simulink model "IRP6"  (R2015a)
settings: Solver=ode1  StartTime=0.0  StopTime=Inf  FixedStep=0.001  RelTol=1e-3
PostLoadFcn:
  | , if any(exist('dsrtsu_mdlpostloadfcn', 'file') == [2, 3, 6]), try dsrtsu_mdlpostloadfcn('Execute', bdroot); catch fprintf('Error in PostLoadFcn (dsrtsu_mdlpostloadfcn) for model "%s":\n %s\n', bdroot, lasterr); end, end,
libraries: simulink x15, rtilibm x3
(part 1 of 2)
settings Model: DSRTSU_INTERNAL_RTI_VER=460  DSRTSU_INTERNAL_RTI_TYPE=rti1005  DSRTSU_INTERNAL_RTIFPGA=50  CovHtmlReporting=off  Creator=k22p800b  LastModifiedBy=k22p800b
settings OptimizationCC: BlockReduction=off  BooleanDataType=off  OptimizeBlockIOStorage=off  BufferReuse=off  GlobalBufferReuse=off  ExpressionFolding=off  LocalBlockOutputs=off
settings HardwareCC: ProdIntDivRoundTo=Zero  ProdEndianess=BigEndian  ProdHWDeviceType=Generic->Custom  TargetIntDivRoundTo=Zero  TargetEndianess=BigEndian  TargetHWDeviceType=Generic->Custom
settings RTWCC: SystemTargetFile=rti1005.tlc  MakeCommand=make_rti  TemplateMakefile=rti1005.tmf  Description=dSPACE DS1005 Hardware Platform
settings STFCustomTargetCC: GenerateSampleERTMain=off  ParMdlRefBuildCompliant=on  GeneratePreprocessorConditionals=Disable all  ERTCustomFileBanners=off  SupportNonInlinedSFcns=on  SupportVariableSizeSignals=off  MATLABClassNameForMDSCustomization=Simulink.SoftwareTarget.GRTCustomization  GRTInterface=on  SystemTargetFile=rti1005.tlc
settings GRTTargetCC: CompOptLevelCompliant=off  ConcurrentExecutionCompliant=off  CombineOutputUpdateFcns=off  MatFileLogging=off  CPPClassGenCompliant=off  GRTInterface=on  ExtModeMexFile=noextcomm

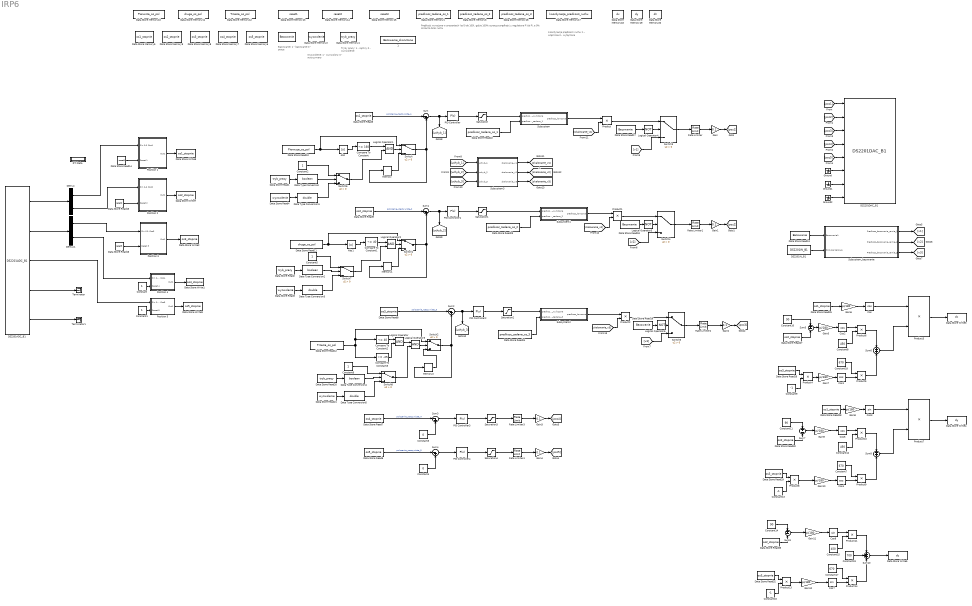
== system IRP6 ==
  note: A
  note: Bazowanie:
      | 1 - bazowanie
      | 0 - praca
  note: Tryby pracy:
      | 1 - ręczny
      | 0 - wyzwolenie
  note: Wyzwolenie:
      | 1 - wyzwolony
      | 0 - wstrzymany
  note: Prędkość wyrażona w procentach (od 0 do 100), gdzie 100% oznacza
      | prędkość z regulatora P lub PI, a 0% oznacza brak ruchu
  note: Koordynacja prędkości ruchu:
      | 1 - włącznoa
      | 0 - wyłączona
  " " : DataStoreMemory  DataStoreName=Bazowanie  ReadBeforeWriteMsg=warning  WriteAfterWriteMsg=warning  WriteAfterReadMsg=warning  OutMin=[0]  OutMax=[1]
  " 1" : DataStoreMemory  DataStoreName=Bazowanie_skonczone  ReadBeforeWriteMsg=warning  WriteAfterWriteMsg=warning  WriteAfterReadMsg=warning  OutMin=[0]  OutMax=[1]
  Abs : Abs
  Abs1 : Abs
  Compare To Constant : simulink/Logic and Bit Operations/Compare To Constant  relop=<=  const=160  OutDataTypeStr=boolean
  Compare To Constant1 : simulink/Logic and Bit Operations/Compare To Constant  relop=<=  const=40  OutDataTypeStr=boolean
  Compare To Constant2 : simulink/Logic and Bit Operations/Compare To Constant  relop=<=  const=40  OutDataTypeStr=boolean
  Compare To Constant3 : simulink/Logic and Bit Operations/Compare To Constant  relop=>=  const=-25  OutDataTypeStr=boolean
  Constant{,1..2,5..6} (5 alike) : Constant
  Constant10 : Constant  Value=90
  Constant11 : Constant  Value=90
  Constant12 : Constant  Value=450
  Constant13 : Constant  Value=-1
  Constant14 : Constant  Value=90
  Constant15 : Constant  Value=450
  Constant16 : Constant  Value=-1
  Constant17 : Constant  Value=670
  Constant18 : Constant  Value=670
  Constant19 : Constant  Value=700
  Constant3 : Constant  Value=0
  Constant4 : Constant  Value=0
  Constant7 : Constant  Value=670
  Constant8 : Constant  Value=450
  Constant9 : Constant  Value=-1
  Cos{,1..2,4..5} (5 alike) : Trigonometry  Operator=cos
  Cos3 : Trigonometry
  Cos7 : Trigonometry
  Cos8 : Trigonometry
  DS2201ADC_B1 : rtilibm/DS2201/DS2201ADC_B1  BoardNo=1  channelNo1=[1 2 3 4]  channelNo2=[5 6 7 8]  channelNo3=[9 10]  channelNo4=-1  channelNo5=-1  DialogFcn=gui2201adc  UnitName={'DS2201ADC_B'}  UnitValues={ 1 }  DSProperties=struct('RTI',struct('Version',uint32(1),'BlockType',struct('isSLSource',uint8(1),'isSLSink',uint8(0),'isHWSource',uint8(1),'isHWSink',uint8(0),'isSetup',uint8(0),'isInline',uint8(1),'isNonInline',uint8(0),'isInterrupt',uint8(0),'isChannelwise',uint8(0)),'IOBoardType','DS2201','UnitType','ADC','Identifier','ADCMUX','DialogType','ML','BlockSet','NONE','SlaveProcessor','NONE'))
  DS2201DAC_B1 : rtilibm/DS2201/DS2201DAC_B1  BoardNo=1  IOErrorMode=[0 0]  InitValue=[0 0 0 0 0 0 0 0]  TermMode=[0 0 0 0 0 0 0 0]  TermValue=[0 0 0 0 0 0 0 0]  DialogFcn=gui2201dac  UnitName={'DS2201DAC_B'}  UnitValues={ 1 }  DSProperties=struct('RTI',struct('Version',uint32(1),'BlockType',struct('isSLSource',uint8(0),'isSLSink',uint8(1),'isHWSource',uint8(0),'isHWSink',uint8(1),'isSetup',uint8(0),'isInline',uint8(1),'isNonInline',uint8(0),'isInterrupt',uint8(0),'isChannelwise',uint8(0)),'IOBoardType','DS2201','UnitType','DAC','Identifier','DAC','DialogType','ML','BlockSet','NONE','SlaveProcessor','NONE'))
  DS2201IN_B1 : rtilibm/DS2201/DS2201IN_B1  BoardNo=1  ChannelNos=[1 2 3]  DialogFcn=gui2201in  UnitName={ 'DS2201IN_B' }  UnitValues={ 1 }  DSProperties=struct('RTI',struct('Version',uint32(1),'BlockType',struct('isSLSource',uint8(1),'isSLSink',uint8(0),'isHWSource',uint8(1),'isHWSink',uint8(0),'isSetup',uint8(0),'isInline',uint8(1),'isNonInline',uint8(0),'isInterrupt',uint8(0),'isChannelwise',uint8(0)),'IOBoardType','DS2201','UnitType','BIT','Identifier','BITIN','DialogType','ML','BlockSet','NONE','SlaveProcessor','NONE'))
  Data Store Memory1 : DataStoreMemory  DataStoreName=predkosc_zadana_os_1  ReadBeforeWriteMsg=warning  WriteAfterWriteMsg=warning  WriteAfterReadMsg=warning  InitialValue=100  OutMin=[0]  OutMax=[100]
  Data Store Memory10 : DataStoreMemory  DataStoreName=Pierwsza_os_pol  ReadBeforeWriteMsg=warning  WriteAfterWriteMsg=warning  WriteAfterReadMsg=warning  OutMin=[-180]  OutMax=[180]
  Data Store Memory11 : DataStoreMemory  DataStoreName=druga_os_pol  ReadBeforeWriteMsg=warning  WriteAfterWriteMsg=warning  WriteAfterReadMsg=warning  OutMin=[-180]  OutMax=[180]
  Data Store Memory12 : DataStoreMemory  DataStoreName=Trzecia_os_pol  ReadBeforeWriteMsg=warning  WriteAfterWriteMsg=warning  WriteAfterReadMsg=warning  OutMin=[-180]  OutMax=[180]
  Data Store Memory13 : DataStoreMemory  DataStoreName=reset1  ReadBeforeWriteMsg=warning  WriteAfterWriteMsg=warning  WriteAfterReadMsg=warning  InitialValue=1  OutMin=[-180]  OutMax=[180]
  Data Store Memory14 : DataStoreMemory  DataStoreName=reset2  ReadBeforeWriteMsg=warning  WriteAfterWriteMsg=warning  WriteAfterReadMsg=warning  InitialValue=1  OutMin=[-180]  OutMax=[180]
  Data Store Memory15 : DataStoreMemory  DataStoreName=reset3  ReadBeforeWriteMsg=warning  WriteAfterWriteMsg=warning  WriteAfterReadMsg=warning  InitialValue=1  OutMin=[-180]  OutMax=[180]
  Data Store Memory16 : DataStoreMemory  DataStoreName=predkosc_zadana_os_3  ReadBeforeWriteMsg=warning  WriteAfterWriteMsg=warning  WriteAfterReadMsg=warning  InitialValue=100  OutMin=[0]  OutMax=[100]
  Data Store Memory17 : DataStoreMemory  DataStoreName=koordynacja_predkosci_ruchu  ReadBeforeWriteMsg=warning  WriteAfterWriteMsg=warning  WriteAfterReadMsg=warning  OutMin=[0]  OutMax=[1]
  Data Store Memory18 : DataStoreMemory  DataStoreName=dx  ReadBeforeWriteMsg=warning  WriteAfterWriteMsg=warning  WriteAfterReadMsg=warning  InitialValue=100  OutMin=[0]  OutMax=[100]
  Data Store Memory19 : DataStoreMemory  DataStoreName=dy  ReadBeforeWriteMsg=warning  WriteAfterWriteMsg=warning  WriteAfterReadMsg=warning  InitialValue=100  OutMin=[0]  OutMax=[100]
  Data Store Memory2 : DataStoreMemory  DataStoreName=wyzwolenie  ReadBeforeWriteMsg=warning  WriteAfterWriteMsg=warning  WriteAfterReadMsg=warning  OutMin=[0]  OutMax=[1]
  Data Store Memory20 : DataStoreMemory  DataStoreName=dz  ReadBeforeWriteMsg=warning  WriteAfterWriteMsg=warning  WriteAfterReadMsg=warning  InitialValue=100  OutMin=[0]  OutMax=[100]
  Data Store Memory3 : DataStoreMemory  DataStoreName=predkosc_zadana_os_2  ReadBeforeWriteMsg=warning  WriteAfterWriteMsg=warning  WriteAfterReadMsg=warning  InitialValue=100  OutMin=[0]  OutMax=[100]
  Data Store Memory4 : DataStoreMemory  DataStoreName=tryb_pracy  ReadBeforeWriteMsg=warning  WriteAfterWriteMsg=warning  WriteAfterReadMsg=warning  InitialValue=1  OutMin=[0]  OutMax=[1]
  Data Store Memory5 : DataStoreMemory  DataStoreName=os1_stopnie  ReadBeforeWriteMsg=warning  WriteAfterWriteMsg=warning  WriteAfterReadMsg=warning
  Data Store Memory6 : DataStoreMemory  DataStoreName=os5_stopnie  ReadBeforeWriteMsg=warning  WriteAfterWriteMsg=warning  WriteAfterReadMsg=warning
  Data Store Memory7 : DataStoreMemory  DataStoreName=os4_stopnie  ReadBeforeWriteMsg=warning  WriteAfterWriteMsg=warning  WriteAfterReadMsg=warning
  Data Store Memory8 : DataStoreMemory  DataStoreName=os3_stopnie  ReadBeforeWriteMsg=warning  WriteAfterWriteMsg=warning  WriteAfterReadMsg=warning
  Data Store Memory9 : DataStoreMemory  DataStoreName=os2_stopnie  ReadBeforeWriteMsg=warning  WriteAfterWriteMsg=warning  WriteAfterReadMsg=warning
  Data Store Read1 : DataStoreRead  DataStoreName=tryb_pracy
  Data Store Read10 : DataStoreRead  DataStoreName=Pierwsza_os_pol
  Data Store Read11 : DataStoreRead  DataStoreName=druga_os_pol
  Data Store Read12 : DataStoreRead  DataStoreName=Trzecia_os_pol
  Data Store Read{13,17..19} (4 alike) : DataStoreRead  DataStoreName=Bazowanie
  Data Store Read14 : DataStoreRead  DataStoreName=reset1
  Data Store Read15 : DataStoreRead  DataStoreName=reset2
  Data Store Read16 : DataStoreRead  DataStoreName=reset3
  Data Store Read2 : DataStoreRead  DataStoreName=tryb_pracy
  Data Store Read20 : DataStoreRead  DataStoreName=tryb_pracy
  Data Store Read21 : DataStoreRead  DataStoreName=wyzwolenie
  Data Store Read22 : DataStoreRead  DataStoreName=predkosc_zadana_os_1
  Data Store Read23 : DataStoreRead  DataStoreName=predkosc_zadana_os_2
  Data Store Read24 : DataStoreRead  DataStoreName=predkosc_zadana_os_3
  Data Store Read25 : DataStoreRead  DataStoreName=os1_stopnie
  Data Store Read{8,26,29,32} (4 alike) : DataStoreRead  DataStoreName=os3_stopnie
  Data Store Read{9,27,30,33} (4 alike) : DataStoreRead  DataStoreName=os2_stopnie
  Data Store Read28 : DataStoreRead  DataStoreName=os1_stopnie
  Data Store Read3 : DataStoreRead  DataStoreName=wyzwolenie
  Data Store Read4 : DataStoreRead  DataStoreName=wyzwolenie
  Data Store Read5 : DataStoreRead  DataStoreName=os1_stopnie
  Data Store Read6 : DataStoreRead  DataStoreName=os5_stopnie
  Data Store Read7 : DataStoreRead  DataStoreName=os4_stopnie
  Data Store Write1 : DataStoreWrite  DataStoreName=os4_stopnie
  Data Store Write2 : DataStoreWrite  DataStoreName=os3_stopnie
  Data Store Write3 : DataStoreWrite  DataStoreName=dx
  Data Store Write4 : DataStoreWrite  DataStoreName=dy
  Data Store Write5 : DataStoreWrite  DataStoreName=dz
  Data Store Write7 : DataStoreWrite  DataStoreName=os2_stopnie
  Data Store Write8 : DataStoreWrite  DataStoreName=os1_stopnie
  Data Store Write9 : DataStoreWrite  DataStoreName=os5_stopnie
  Data Type Conversion : DataTypeConversion  OutDataTypeStr=boolean
  Data Type Conversion1 : DataTypeConversion  OutDataTypeStr=double
  Data Type Conversion2 : DataTypeConversion  OutDataTypeStr=boolean
  Data Type Conversion3 : DataTypeConversion  OutDataTypeStr=double
  Data Type Conversion4 : DataTypeConversion  OutDataTypeStr=boolean
  Data Type Conversion5 : DataTypeConversion  OutDataTypeStr=double
  Demux : Demux  Outputs=2
  Demux1 : Demux  Outputs=2
  Gain{,1..4} (5 alike) : Gain  Gain=0.1
  Gain{5..12} (8 alike) : Gain  Gain=pi/180
  Ground : Ground
  Ground1 : Ground
  Ground2 : Ground
  Logical Operator{,1..3} (4 alike) : Logic  AllPortsSameDT=off
  Logical Operator4 : Logic  Operator=NOT  AllPortsSameDT=off
  Logical Operator5 : Logic  Operator=NOT  AllPortsSameDT=off
  Logical Operator6 : Logic  Operator=NOT  AllPortsSameDT=off
  Memory : Memory
  Memory1 : Memory
  Memory2 : Memory
  PID Controller{,1..4} (5 alike) : simulink/Continuous/PID Controller  Controller=P  TimeDomain=Continuous-time  SampleTime=-1  IntegratorMethod=Forward Euler  FilterMethod=Forward Euler  Form=Parallel  UseFilter=on  ControllerParametersSource=internal  P=0.5  I=0  D=0  N=100  InitialConditionSource=internal  InitialConditionForIntegrator=0  InitialConditionForFilter=0  ExternalReset=none  LimitOutput=off  UpperSaturationLimit=inf  LowerSaturationLimit=-inf  LinearizeAsGain=on  AntiWindupMode=none  Kb=1  TrackingMode=off  Kt=1  PParamMin=[]  PParamMax=[]  IParamMin=[]  IParamMax=[]  DParamMin=[]  DParamMax=[]  NParamMin=[]  NParamMax=[]  KbParamMin=[]  KbParamMax=[]  KtParamMin=[]  KtParamMax=[]  POutMin=[]  POutMax=[]  IOutMin=[]  IOutMax=[]  DOutMin=[]  DOutMax=[]  NOutMin=[]  NOutMax=[]  KbOutMin=[]  KbOutMax=[]  KtOutMin=[]  KtOutMax=[]  IntegratorOutMin=[]  IntegratorOutMax=[]  FilterOutMin=[]  FilterOutMax=[]  SumOutMin=[]  SumOutMax=[]  SumI1OutMin=[]  SumI1OutMax=[]  SumI2OutMin=[]  SumI2OutMax=[]  SumI3OutMin=[]  SumI3OutMax=[]  SumDOutMin=[]  SumDOutMax=[]  SaturationOutMin=[]  SaturationOutMax=[]  IntegratorContinuousStateAttributes=''  IntegratorStateMustResolveToSignalObject=off  IntegratorRTWStateStorageClass=Auto  FilterContinuousStateAttributes=''  FilterStateMustResolveToSignalObject=off  FilterRTWStateStorageClass=Auto  DifferentiatorICPrevScaledInput=0  DifferentiatorOutMin=[]  DifferentiatorOutMax=[]
  Position 1 : Subsystem
  Position 2 : Subsystem
  Position 3 : Subsystem
  Position 4 : Subsystem
  Position 5 : Subsystem
  Product{,1..11,13..14} (14 alike) : Product
  RTI Data : Subsystem  Tag=struct('RTIDataServer',struct('RTIDataServerVs','2','RTIModelDescription','struct(''main'',''FANUC_2015a'',''sub'','''',''isMp'',0)'))  LoadFcn="if exist('rtidc'), try,  rtidc('DataHostBlockClbLoad', gcbh); catch, disp(['Warning: ''LoadFcn'' for RTI Data block failed: ' lasterr]); end, end,"  mask(RTI_DATA_HOST){}
      mask help:
      | RTI Data Block.
      | This block is used by RTI to store internal model-dependent data.
      | Please keep this block on the root level of the model. Deleting this block will result in data loss.
      |
      | NEVER DELETE OR COPY THIS BLOCK!
      settings: CopyFcn="if exist('rtidc'), try,  rtidc('DataHostBlockClbCopy', gcbh); catch, disp(['Warning: ''CopyFcn'' for RTI Data block failed: ' lasterr]); end, end,"  DeleteFcn="if exist('rtidc'), try,  rtidc('DataHostBlockClbDelete', gcbh); catch, disp(['Warning: ''DeleteFcn'' for RTI Data block failed: ' lasterr]); end, end,"  ModelCloseFcn="if exist('rtidc'), try,  rtidc('DataHostBlockClbModelClose', gcbh); catch, disp(['Warning: ''ModelCloseFcn'' for RTI Data block failed: ' lasterr]); end, end,"  PreSaveFcn="if exist('rtidc'), try,  rtidc('DataHostBlockClbPreSave', gcbh); catch, disp(['Warning: ''PreSaveFcn'' for RTI Data block failed: ' lasterr]); end, end,"  PostSaveFcn="if exist('rtidc'), try,  rtidc('DataHostBlockClbPostSave', gcbh); catch, disp(['Warning: ''PostSaveFcn'' for RTI Data block failed: ' lasterr]); end, end,"  NameChangeFcn="if exist('rtidc'), try,  rtidc('DataHostBlockClbNameChange', gcbh); catch, disp(['Warning: ''NameChangeFcn'' for RTI Data block failed: ' lasterr]); end, end,"
      mask Help:
      | RTI Data Block.
      | This block is used by RTI to store internal model-dependent data.
      | Please keep this block on the root level of the model. Deleting this block will result in data loss.
      | 
      | NEVER DELETE OR COPY THIS BLOCK!
      mask Display:
      | text(0.5, 0.5, 'RTI Data', 'HorizontalAlignment', 'center');
      | plot([1 0]);
  Rate Limiter{,1..4} (5 alike) : RateLimiter  RisingSlewLimit=50  FallingSlewLimit=-50  SampleTimeMode=inherited
  Saturation{,1..4} (5 alike) : Saturate  UpperLimit=3  LowerLimit=-3
  Subsystem : Subsystem
  Subsystem1 : Subsystem
  Subsystem2 : Subsystem
  Subsystem3 : Subsystem
  Subsystem_bazowanie : Subsystem
  Sum{,1..4} (5 alike) : Sum  Inputs=|-+
  Sum10 : Sum  Inputs=+++
  Sum5 : Sum  Inputs=+-
  Sum6 : Sum
  Sum7 : Sum  Inputs=+-
  Sum8 : Sum
  Sum9 : Sum  Inputs=+-
  Switch{,1..8} (9 alike) : Switch  Criteria=u2 > Threshold
  Terminator : Terminator
  Terminator1 : Terminator
  wires:
  DS2201ADC_B1/1 -> Demux/1
  DS2201ADC_B1/2 -> Demux1/1
  DS2201ADC_B1/4 -> Terminator/1
  DS2201ADC_B1/5 -> Terminator1/1
  Demux/1 -> Position 1/1(Sin && Cos1)
  Demux1/1 -> Position 3/1(Sin && Cos3)
  Demux1/2 -> Position 4/1(Sin && Cos4)
  DS2201ADC_B1/3 -> Position 5/1(Sin && Cos5)
  Demux/2 -> Position 2/1(Sin && Cos2)
  Position 2/1(Out1) -> Data Store Write7/1
  Position 4/1(Out1) -> Data Store Write1/1
  Position 3/1(Out1) -> Data Store Write2/1
  Position 5/1(Out1) -> Data Store Write9/1
  Position 1/1(Out1) -> Data Store Write8/1
  Data Store Read5/1 -> Sum/1  "polozenie_rzeczywiste_1"
  Sum/1 -> [uchyb_1], PID Controller/1
  PID Controller/1 -> Saturation/1
  Rate Limiter/1 -> Gain/1
  Gain/1 -> [poz1]
  [poz1] -> DS2201DAC_B1/1
  Data Store Read9/1 -> Sum1/1  "polozenie_rzeczywiste_2"
  Sum1/1 -> [uchyb_2], PID Controller1/1
  PID Controller1/1 -> Saturation1/1
  Rate Limiter1/1 -> Gain1/1
  Gain1/1 -> [poz2]
  [poz2] -> DS2201DAC_B1/2
  [poz4] -> DS2201DAC_B1/4
  [poz5] -> DS2201DAC_B1/5
  [poz3] -> DS2201DAC_B1/3
  Data Store Read8/1 -> Sum2/1  "polozenie_rzeczywiste_3"
  Sum2/1 -> [uchyb_3], PID Controller2/1
  PID Controller2/1 -> Saturation2/1
  Rate Limiter2/1 -> Gain2/1
  Gain2/1 -> [poz3]
  Data Store Read7/1 -> Sum3/1  "polozenie_rzeczywiste_4"
  Sum3/1 -> PID Controller3/1
  PID Controller3/1 -> Saturation3/1
  Saturation3/1 -> Rate Limiter3/1
  Constant3/1 -> Sum3/2
  Rate Limiter3/1 -> Gain3/1
  Gain3/1 -> [poz4]
  Data Store Read6/1 -> Sum4/1  "polozenie_rzeczywiste_5"
  Sum4/1 -> PID Controller4/1
  PID Controller4/1 -> Saturation4/1
  Saturation4/1 -> Rate Limiter4/1
  Constant4/1 -> Sum4/2
  Rate Limiter4/1 -> Gain4/1
  Gain4/1 -> [poz5]
  Data Store Read10/1 -> Switch/1, Abs/1
  Memory/1 -> Switch/3
  Switch/1 -> Sum/2, Memory/1
  Abs/1 -> Compare To Constant/1
  Data Store Read11/1 -> Switch1/1, Abs1/1
  Memory1/1 -> Switch1/3
  Switch1/1 -> Memory1/1, Sum1/2
  Abs1/1 -> Compare To Constant1/1
  Memory2/1 -> Switch2/3
  Switch2/1 -> Memory2/1, Sum2/2
  Data Store Read12/1 -> Compare To Constant3/1, Compare To Constant2/1, Switch2/1
  Compare To Constant2/1 -> Logical Operator/1
  Compare To Constant3/1 -> Logical Operator/2
  Ground2/1 -> DS2201DAC_B1/8
  Ground1/1 -> DS2201DAC_B1/7
  Ground/1 -> DS2201DAC_B1/6
  DS2201IN_B1/1 -> Subsystem_bazowanie/2("Pozycja bazowa ")
  Subsystem_bazowanie/1(Predkosc_bazowania_ramie_1) -> [v1]
  Subsystem_bazowanie/2(Predkosc_bazowania_ramie_2) -> [v2]
  Data Store Read14/1 -> Position 1/2(Reset 1)
  Data Store Read15/1 -> Position 2/2(Reset 2)
  Data Store Read16/1 -> Position 3/2(Reset 3)
  Switch3/1 -> Rate Limiter/1
  Subsystem_bazowanie/3(Predkosc_bazowania_ramie_3) -> [v3]
  [v1] -> Switch3/3
  [v2] -> Switch4/3
  Switch4/1 -> Rate Limiter1/1
  [v3] -> Switch5/3
  Switch5/1 -> Rate Limiter2/1
  Constant/1 -> Position 4/2(Reset 4)
  Constant1/1 -> Position 5/2(Reset 5)
  Data Store Read4/1 -> Data Type Conversion1/1
  Data Type Conversion/1 -> Switch6/2
  Data Type Conversion1/1 -> Switch6/3
  Data Store Read1/1 -> Data Type Conversion/1
  Constant2/1 -> Switch6/1
  Logical Operator1/1 -> Switch/2
  Compare To Constant/1 -> Logical Operator1/1
  Switch6/1 -> Logical Operator1/2
  Constant5/1 -> Switch7/1
  Data Type Conversion2/1 -> Switch7/2
  Data Type Conversion3/1 -> Switch7/3
  Data Store Read2/1 -> Data Type Conversion2/1
  Data Store Read3/1 -> Data Type Conversion3/1
  Constant6/1 -> Switch8/1
  Data Type Conversion4/1 -> Switch8/2
  Data Type Conversion5/1 -> Switch8/3
  Data Store Read20/1 -> Data Type Conversion4/1
  Data Store Read21/1 -> Data Type Conversion5/1
  Logical Operator2/1 -> Switch1/2
  Compare To Constant1/1 -> Logical Operator2/1
  Switch7/1 -> Logical Operator2/2
  Logical Operator3/1 -> Switch2/2
  Logical Operator/1 -> Logical Operator3/1
  Switch8/1 -> Logical Operator3/2
  Data Store Read22/1 -> Subsystem/2(predkosc_zadana_1)
  Saturation/1 -> Subsystem/1(predkosc_wyliczona)
  Data Store Read23/1 -> Subsystem1/2(predkosc_zadana_2)
  Saturation1/1 -> Subsystem1/1(predkosc_wyliczona)
  Data Store Read24/1 -> Subsystem2/2(predkosc_zadana_3)
  Saturation2/1 -> Subsystem2/1(predkosc_wyliczona)
  [uchyb_1] -> Subsystem3/1(uchyb_1)
  [uchyb_2] -> Subsystem3/2(uchyb_2)
  [uchyb_3] -> Subsystem3/3(uchyb_3)
  Subsystem/1(predkosc_koncowa) -> Product/1
  Product/1 -> Switch3/1
  Subsystem3/1(skalowanie_v1) -> [skalowanie_v1]
  Subsystem3/2(skalowanie_v2) -> [skalowanie_v2]
  Subsystem3/3(skalowanie_v3) -> [skalowanie_v3]
  [skalowanie_v1] -> Product/2
  [skalowanie_v2] -> Product1/2
  Subsystem1/1(predkosc_koncowa) -> Product1/1
  [skalowanie_v3] -> Product2/2
  Subsystem2/1(predkosc_koncowa) -> Product2/1
  Product2/1 -> Switch5/1
  Product1/1 -> Switch4/1
  Data Store Read25/1 -> Gain6/1
  Cos/1 -> Product3/1
  Product4/1 -> Gain7/1
  Data Store Read26/1 -> Product4/1
  Constant9/1 -> Product4/2
  Cos1/1 -> Product5/2
  Constant10/1 -> Sum5/1
  Data Store Read27/1 -> Sum5/2
  Sum5/1 -> Gain5/1
  Cos2/1 -> Product6/1
  Constant8/1 -> Product6/2
  Product5/1 -> Sum6/2
  Product6/1 -> Sum6/1
  Sum6/1 -> Product3/2
  Product3/1 -> Data Store Write3/1
  Product10/1 -> Sum8/1
  Product8/1 -> Gain10/1
  Product9/1 -> Sum8/2
  Product7/1 -> Data Store Write4/1
  Data Store Read28/1 -> Gain8/1
  Constant13/1 -> Product8/2
  Sum7/1 -> Gain9/1
  Data Store Read30/1 -> Sum7/2
  Cos3/1 -> Product7/1
  Cos5/1 -> Product10/1
  Constant12/1 -> Product10/2
  Data Store Read29/1 -> Product8/1
  Constant11/1 -> Sum7/1
  Cos4/1 -> Product9/2
  Sum8/1 -> Product7/2
  Data Store Read32/1 -> Product13/1
  Constant14/1 -> Sum9/1
  Constant15/1 -> Product11/2
  Cos7/1 -> Product14/2
  Sum9/1 -> Gain11/1
  Constant16/1 -> Product13/2
  Cos8/1 -> Product11/1
  Data Store Read33/1 -> Sum9/2
  Sum10/1 -> Data Store Write5/1
  Product13/1 -> Gain12/1
  Product11/1 -> Sum10/1
  Constant7/1 -> Product9/1
  Constant17/1 -> Product14/1
  Constant18/1 -> Product5/1
  Product14/1 -> Sum10/3
  Constant19/1 -> Sum10/2
  Data Store Read17/1 -> Logical Operator4/1
  Logical Operator4/1 -> Switch3/2
  Data Store Read18/1 -> Logical Operator5/1
  Logical Operator5/1 -> Switch4/2
  Data Store Read19/1 -> Logical Operator6/1
  Logical Operator6/1 -> Switch5/2
  Data Store Read13/1 -> Subsystem_bazowanie/1(Bazowanie1)
  Gain5/1 -> Cos2/1
  Gain6/1 -> Cos/1
  Gain7/1 -> Cos1/1
  Gain8/1 -> Cos3/1
  Gain9/1 -> Cos5/1
  Gain10/1 -> Cos4/1
  Gain11/1 -> Cos8/1
  Gain12/1 -> Cos7/1

== system IRP6/Position 1 ==
  Sin && Cos1 : Inport
  Reset 1 : Inport  Port=2
  Filters 1 : Subsystem
  Position Calculation 1 : Subsystem
  Out1 : Outport
  wires:
  Position Calculation 1/1(Position) -> Out1/1
  Reset 1/1 -> Position Calculation 1/3(Reset (Impulse))
  Sin && Cos1/1 -> Filters 1/1(Sin && Cos)
  Filters 1/2(Cos) -> Position Calculation 1/2(Cos)
  Filters 1/1(Sin) -> Position Calculation 1/1(Sin)

== system IRP6/Position 2 ==
  Sin && Cos2 : Inport
  Reset 2 : Inport  Port=2
  Filters 2 : Subsystem
  Position Calculation 2 : Subsystem
  Out1 : Outport
  wires:
  Position Calculation 2/1(Position) -> Out1/1
  Reset 2/1 -> Position Calculation 2/3(Reset (Impulse))
  Sin && Cos2/1 -> Filters 2/1(Sin && Cos)
  Filters 2/2(Cos) -> Position Calculation 2/2(Cos)
  Filters 2/1(Sin) -> Position Calculation 2/1(Sin)

== system IRP6/Position 3 ==
  Sin && Cos3 : Inport
  Reset 3 : Inport  Port=2
  Filters 3 : Subsystem
  Position Calculation 3 : Subsystem
  Out1 : Outport
  wires:
  Position Calculation 3/1(Position) -> Out1/1
  Reset 3/1 -> Position Calculation 3/3(Reset (Impulse))
  Sin && Cos3/1 -> Filters 3/1(Sin && Cos)
  Filters 3/2(Cos) -> Position Calculation 3/2(Cos)
  Filters 3/1(Sin) -> Position Calculation 3/1(Sin)

== system IRP6/Position 4 ==
  Sin && Cos4 : Inport
  Reset 4 : Inport  Port=2
  Filters 4 : Subsystem
  Position Calculation 4 : Subsystem
  Out1 : Outport
  wires:
  Filters 4/1(Sin) -> Position Calculation 4/1(Sin)
  Filters 4/2(Cos) -> Position Calculation 4/2(Cos)
  Sin && Cos4/1 -> Filters 4/1(Sin && Cos)
  Reset 4/1 -> Position Calculation 4/3(Reset (Impulse))
  Position Calculation 4/1(Position) -> Out1/1

== system IRP6/Position 5 ==
  Sin && Cos5 : Inport
  Reset 5 : Inport  Port=2
  Filters 5 : Subsystem
  Position Calculation 5 : Subsystem
  Out1 : Outport
  wires:
  Filters 5/1(Sin) -> Position Calculation 5/1(Sin)
  Filters 5/2(Cos) -> Position Calculation 5/2(Cos)
  Sin && Cos5/1 -> Filters 5/1(Sin && Cos)
  Reset 5/1 -> Position Calculation 5/3(Reset (Impulse))
  Position Calculation 5/1(Position) -> Out1/1

== system IRP6/RTI Data ==
  RTI Data Store : Subsystem  Tag="struct('private',struct('version',struct('dsVer',uint32(2),'dsVerCreation',uint32(2),'RTI',struct('ver','7.4','type','RTI1005')),'access',struct('type','Model','isPerm',1,'created',['05-Dec-2022 09:12:52'],'modified',['12-Dec-2022 09:25:57'],'location','')),'public',struct('main',struct('data',[]),'sub',struct('name',{{'FANUC_2015a'}},'data',{{struct('TH',struct('thTaskInfo',struct('taskType',{'TIMER','HWINT','TMRINT','SWINT','GLINT'},'tasksNumOf',{1,0,0,0,0},'srcIds',{{'TIMERA'},{},{},{},{}},'taskNames',{{['Timer Task 1']},{},{},{},{}})),'th_tc',struct('dataType','TASK','taskGroupId','','taskGroupList',{{}},'taskSchedulingPolicy','FCFS','taskType','TIMER','blkh',-1,'srcId','TIMERA','srcSgnName',['Timer A interrupt'],'srcCpuName','','taskName',['Timer Task 1  [0.001] s'],'taskNameDisplayExt','','smplTime',0.001,'smplTimeOffs',0,'hasFixedPriority',0,'priority',1,'hasFixedOvc',0,'ovcType',1,'ovcMax',1),'tc_th',struct('dataType','TASK','taskGroupId','','taskGroupList',{{}},'taskSchedulingPolicy','FCFS','taskType','TIMER','blkh',-1,'srcId','TIMERA','srcSgnName',['Timer A interrupt'],'srcCpuName','','taskName',['Timer Task 1  [0.001] s'],'taskNameDisplayExt','','smplTime',0.001,'smplTimeOffs',0,'hasFixedPriority',0,'priority',1,'hasFixedOvc',0,'ovcType',1,'ovcMax',1))}})))"  mask(RTI_DATA_STORE){}
      mask help:
      | RTI Data Store Block. This block is used by RTI to store internal model dependent data. Deleting this block will result in data loss.
      |
      | NEVER DELETE, COPY, OR MODIFY THIS BLOCK!
      mask Help:
      | RTI Data Store Block. This block is used by RTI to store internal model dependent data. Deleting this block will result in data loss.
      | 
      | NEVER DELETE, COPY, OR MODIFY THIS BLOCK!
      mask Display: text(0.5, 0.5, ' ', 'HorizontalAlignment', 'center');

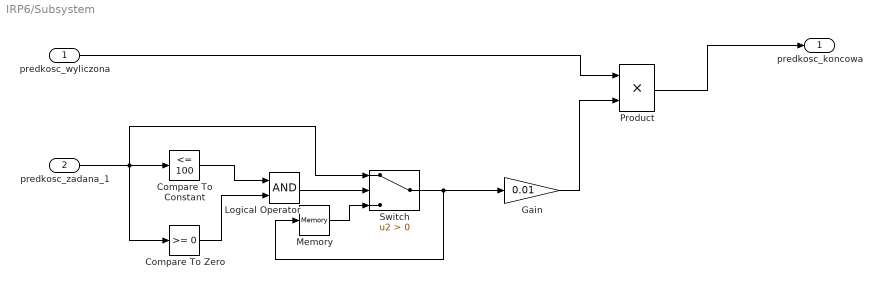
== system IRP6/Subsystem ==
  predkosc_wyliczona : Inport
  predkosc_zadana_1 : Inport  Port=2
  Compare To Constant : simulink/Logic and Bit Operations/Compare To Constant  relop=<=  const=100  OutDataTypeStr=boolean
  Compare To Zero : simulink/Logic and Bit Operations/Compare To Zero  relop=>=  OutDataTypeStr=boolean
  Gain : Gain  Gain=0.01
  Logical Operator : Logic  AllPortsSameDT=off
  Memory : Memory  X0=100
  Product : Product
  Switch : Switch  Criteria=u2 > Threshold
  predkosc_koncowa : Outport
  wires:
  Product/1 -> predkosc_koncowa/1
  predkosc_wyliczona/1 -> Product/1
  predkosc_zadana_1/1 -> Compare To Zero/1, Switch/1, Compare To Constant/1
  Logical Operator/1 -> Switch/2
  Compare To Constant/1 -> Logical Operator/1
  Compare To Zero/1 -> Logical Operator/2
  Memory/1 -> Switch/3
  Switch/1 -> Gain/1, Memory/1
  Gain/1 -> Product/2

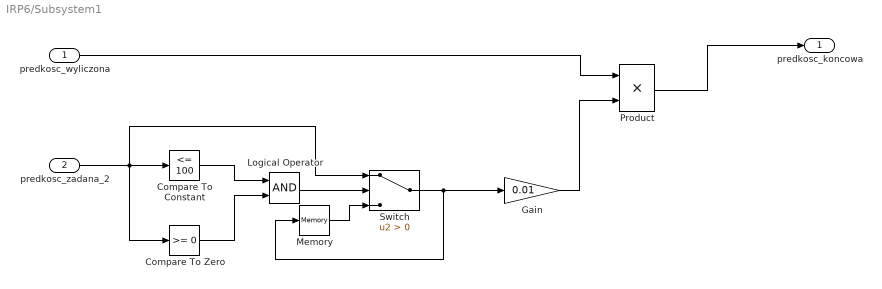
== system IRP6/Subsystem1 ==
  predkosc_wyliczona : Inport
  predkosc_zadana_2 : Inport  Port=2
  Compare To Constant : simulink/Logic and Bit Operations/Compare To Constant  relop=<=  const=100  OutDataTypeStr=boolean
  Compare To Zero : simulink/Logic and Bit Operations/Compare To Zero  relop=>=  OutDataTypeStr=boolean
  Gain : Gain  Gain=0.01
  Logical Operator : Logic  AllPortsSameDT=off
  Memory : Memory  X0=100
  Product : Product
  Switch : Switch  Criteria=u2 > Threshold
  predkosc_koncowa : Outport
  wires:
  Product/1 -> predkosc_koncowa/1
  predkosc_wyliczona/1 -> Product/1
  predkosc_zadana_2/1 -> Compare To Zero/1, Switch/1, Compare To Constant/1
  Logical Operator/1 -> Switch/2
  Compare To Constant/1 -> Logical Operator/1
  Compare To Zero/1 -> Logical Operator/2
  Memory/1 -> Switch/3
  Switch/1 -> Gain/1, Memory/1
  Gain/1 -> Product/2

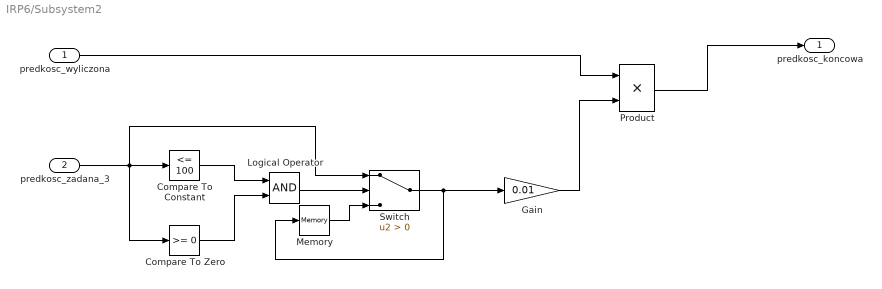
== system IRP6/Subsystem2 ==
  predkosc_wyliczona : Inport
  predkosc_zadana_3 : Inport  Port=2
  Compare To Constant : simulink/Logic and Bit Operations/Compare To Constant  relop=<=  const=100  OutDataTypeStr=boolean
  Compare To Zero : simulink/Logic and Bit Operations/Compare To Zero  relop=>=  OutDataTypeStr=boolean
  Gain : Gain  Gain=0.01
  Logical Operator : Logic  AllPortsSameDT=off
  Memory : Memory  X0=100
  Product : Product
  Switch : Switch  Criteria=u2 > Threshold
  predkosc_koncowa : Outport
  wires:
  Product/1 -> predkosc_koncowa/1
  predkosc_wyliczona/1 -> Product/1
  predkosc_zadana_3/1 -> Compare To Zero/1, Switch/1, Compare To Constant/1
  Logical Operator/1 -> Switch/2
  Compare To Constant/1 -> Logical Operator/1
  Compare To Zero/1 -> Logical Operator/2
  Memory/1 -> Switch/3
  Switch/1 -> Gain/1, Memory/1
  Gain/1 -> Product/2

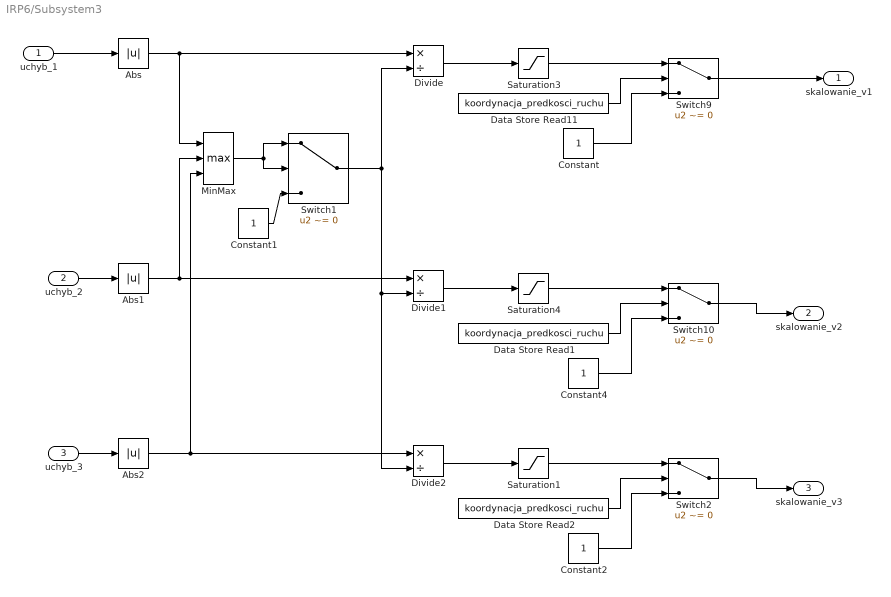
== system IRP6/Subsystem3 ==
  uchyb_1 : Inport
  uchyb_2 : Inport  Port=2
  uchyb_3 : Inport  Port=3
  Abs : Abs
  Abs1 : Abs
  Abs2 : Abs
  Constant{,1..2,4} (4 alike) : Constant
  Data Store Read1 : DataStoreRead  DataStoreName=koordynacja_predkosci_ruchu
  Data Store Read11 : DataStoreRead  DataStoreName=koordynacja_predkosci_ruchu
  Data Store Read2 : DataStoreRead  DataStoreName=koordynacja_predkosci_ruchu
  Divide : Product  Inputs=*/
  Divide1 : Product  Inputs=*/
  Divide2 : Product  Inputs=*/
  MinMax : MinMax  Function=max  Inputs=3
  Saturation1 : Saturate  UpperLimit=1  LowerLimit=0.001
  Saturation3 : Saturate  UpperLimit=1  LowerLimit=0.001
  Saturation4 : Saturate  UpperLimit=1  LowerLimit=0.001
  Switch{1..2,9..10} (4 alike) : Switch  Criteria=u2 ~= 0
  skalowanie_v1 : Outport
  skalowanie_v2 : Outport  Port=2
  skalowanie_v3 : Outport  Port=3
  wires:
  Saturation4/1 -> Switch10/1
  Abs/1 -> Divide/1, MinMax/1
  Switch9/1 -> skalowanie_v1/1
  Constant/1 -> Switch9/3
  Switch10/1 -> skalowanie_v2/1
  Constant4/1 -> Switch10/3
  Divide/1 -> Saturation3/1
  Divide1/1 -> Saturation4/1
  Saturation3/1 -> Switch9/1
  uchyb_1/1 -> Abs/1
  uchyb_2/1 -> Abs1/1
  Data Store Read11/1 -> Switch9/2
  Abs1/1 -> Divide1/1, MinMax/2
  MinMax/1 -> Switch1/2, Switch1/1
  Constant1/1 -> Switch1/3
  Switch1/1 -> Divide/2, Divide2/2, Divide1/2
  Data Store Read1/1 -> Switch10/2
  Abs2/1 -> Divide2/1, MinMax/3
  Data Store Read2/1 -> Switch2/2
  uchyb_3/1 -> Abs2/1
  Saturation1/1 -> Switch2/1
  Switch2/1 -> skalowanie_v3/1
  Divide2/1 -> Saturation1/1
  Constant2/1 -> Switch2/3

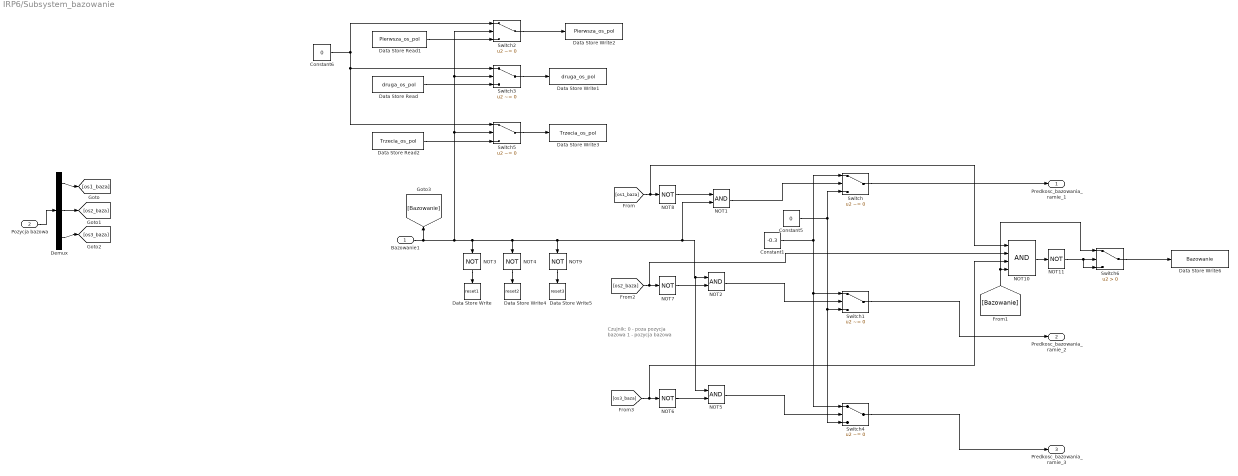
== system IRP6/Subsystem_bazowanie ==
  note: Czujnik:
      | 0 - poza pozycja bazowa
      | 1 - pozycja bazowa
  Bazowanie1 : Inport
  "Pozycja bazowa " : Inport  Port=2
  Constant1 : Constant  Value=-0.3
  Constant5 : Constant  Value=0
  Constant6 : Constant  Value=0
  Data Store Read : DataStoreRead  DataStoreName=druga_os_pol
  Data Store Read1 : DataStoreRead  DataStoreName=Pierwsza_os_pol
  Data Store Read2 : DataStoreRead  DataStoreName=Trzecia_os_pol
  Data Store Write : DataStoreWrite  DataStoreName=reset1
  Data Store Write1 : DataStoreWrite  DataStoreName=druga_os_pol
  Data Store Write2 : DataStoreWrite  DataStoreName=Pierwsza_os_pol
  Data Store Write3 : DataStoreWrite  DataStoreName=Trzecia_os_pol
  Data Store Write4 : DataStoreWrite  DataStoreName=reset2
  Data Store Write5 : DataStoreWrite  DataStoreName=reset3
  Data Store Write6 : DataStoreWrite  DataStoreName=Bazowanie
  Demux : Demux  Outputs=3
  NOT1 : Logic  AllPortsSameDT=off
  NOT10 : Logic  Inputs=4  AllPortsSameDT=off
  NOT{6..8,11} (4 alike) : Logic  Operator=NOT  AllPortsSameDT=off
  NOT2 : Logic  AllPortsSameDT=off
  NOT3 : Logic  Operator=NOT  IconShape=distinctive  AllPortsSameDT=off
  NOT4 : Logic  Operator=NOT  IconShape=distinctive  AllPortsSameDT=off
  NOT5 : Logic  AllPortsSameDT=off
  NOT9 : Logic  Operator=NOT  IconShape=distinctive  AllPortsSameDT=off
  Switch{,1..5} (6 alike) : Switch  Criteria=u2 ~= 0
  Switch6 : Switch  Criteria=u2 > Threshold
  Predkosc_bazowania_ramie_1 : Outport
  Predkosc_bazowania_ramie_2 : Outport  Port=2
  Predkosc_bazowania_ramie_3 : Outport  Port=3
  wires:
  Switch3/1 -> Data Store Write1/1
  Switch1/1 -> Predkosc_bazowania_ramie_2/1
  Switch2/1 -> Data Store Write2/1
  Data Store Read1/1 -> Switch2/3
  NOT2/1 -> Switch1/2
  Data Store Read/1 -> Switch3/3
  Constant1/1 -> Switch4/1, Switch1/1, Switch/1
  Constant6/1 -> Switch2/1, Switch3/1, Switch5/1
  Switch/1 -> Predkosc_bazowania_ramie_1/1
  Bazowanie1/1 -> [Bazowanie], NOT9/1, NOT5/1, NOT2/1, NOT1/2, NOT4/1, NOT3/1, Switch5/2, Switch3/2, Switch2/2
  NOT1/1 -> Switch/2
  Constant5/1 -> Switch4/3, Switch1/3, Switch/3
  "Pozycja bazowa "/1 -> Demux/1
  Demux/3 -> [os3_baza]
  Demux/2 -> [os2_baza]
  Demux/1 -> [os1_baza]
  Switch4/1 -> Predkosc_bazowania_ramie_3/1
  NOT5/1 -> Switch4/2
  [os3_baza] -> NOT10/3, NOT6/1
  NOT6/1 -> NOT5/2
  [os2_baza] -> NOT10/2, NOT7/1
  NOT7/1 -> NOT2/2
  [os1_baza] -> NOT10/1, NOT8/1
  NOT8/1 -> NOT1/1
  Switch5/1 -> Data Store Write3/1
  Data Store Read2/1 -> Switch5/3
  NOT4/1 -> Data Store Write4/1
  NOT9/1 -> Data Store Write5/1
  NOT3/1 -> Data Store Write/1
  NOT10/1 -> NOT11/1
  [Bazowanie] -> Switch6/1, NOT10/4
  NOT11/1 -> Switch6/3, Switch6/2
  Switch6/1 -> Data Store Write6/1

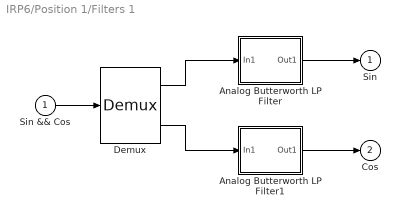
== system IRP6/Position 1/Filters 1 ==
  Sin && Cos : Inport
  Analog Butterworth LP Filter : Subsystem  mask(buttap){Parameter1=2*pi*16, Parameter2=1}
      mask prompts: Parameter1 "Cutoff frequency (rad/sec)"; Parameter2 "Order"
      mask help:
      | Analog Butterworth low pass filter.
      |
      | (Requires Signal Processing Toolbox)
      mask init:
      | [z,p,k]=buttap(@2); z=@1*z; p=@1*p; k=real(prod(-p)); [num,den]=zp2tf(z,p,k); w=logspace(log10(@1/10),log10(10*@1),20); h=freqs(num,den,w);
      mask Help: Butterworth low pass filter using MATLAB's butter command.
      mask Display: plot(20*log10(w),20*log10(abs(h)))
  Analog Butterworth LP Filter1 : Subsystem  mask(buttap){Parameter1=2*pi*16, Parameter2=1}
      mask prompts: Parameter1 "Cutoff frequency (rad/sec)"; Parameter2 "Order"
      mask help:
      | Analog Butterworth low pass filter.
      |
      | (Requires Signal Processing Toolbox)
      mask init:
      | [z,p,k]=buttap(@2); z=@1*z; p=@1*p; k=real(prod(-p)); [num,den]=zp2tf(z,p,k); w=logspace(log10(@1/10),log10(10*@1),20); h=freqs(num,den,w);
      mask Help: Butterworth low pass filter using MATLAB's butter command.
      mask Display: plot(20*log10(w),20*log10(abs(h)))
  Demux : Demux  Outputs=2
  Sin : Outport
  Cos : Outport  Port=2
  wires:
  Analog Butterworth LP Filter/1(Out1) -> Sin/1
  Analog Butterworth LP Filter1/1(Out1) -> Cos/1
  Sin && Cos/1 -> Demux/1
  Demux/1 -> Analog Butterworth LP Filter/1(In1)
  Demux/2 -> Analog Butterworth LP Filter1/1(In1)

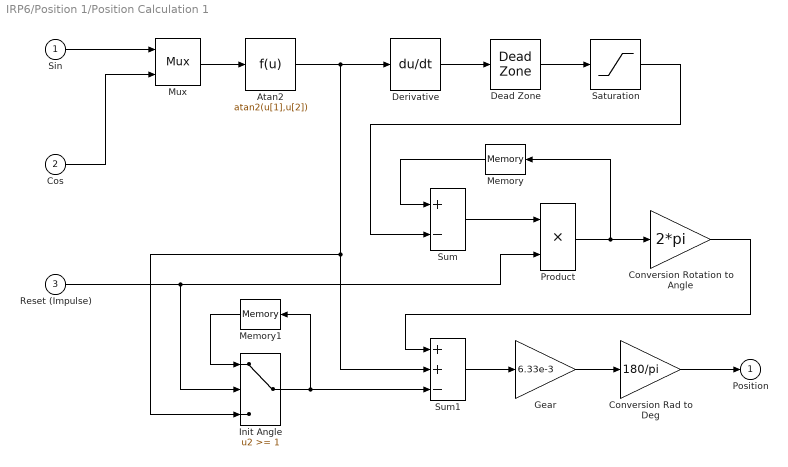
== system IRP6/Position 1/Position Calculation 1 ==
  Sin : Inport
  Cos : Inport  Port=2
  Reset (Impulse) : Inport  Port=3
  Atan2 : Fcn  Expr=atan2(u[1],u[2])
  Conversion Rad to Deg : Gain  Gain=180/pi  SaturateOnIntegerOverflow=on  OutDataTypeStr=Inherit: Same as input  ParamDataTypeStr=Inherit: Same as input
  Conversion Rotation to Angle : Gain  Gain=2*pi  SaturateOnIntegerOverflow=on  OutDataTypeStr=Inherit: Same as input  ParamDataTypeStr=Inherit: Same as input
  Dead Zone : DeadZone  LowerValue=-5000  UpperValue=5000  SaturateOnIntegerOverflow=on
  Derivative : Derivative
  Gear : Gain  Gain=6.33e-3  SaturateOnIntegerOverflow=on  OutDataTypeStr=Inherit: Same as input  ParamDataTypeStr=Inherit: Same as input
  Init Angle : Switch  Threshold=1  SaturateOnIntegerOverflow=on  InputSameDT=on
  Memory : Memory
  Memory1 : Memory
  Mux : Mux  Inputs=2
  Product : Product  SaturateOnIntegerOverflow=on  RndMeth=Zero  InputSameDT=on  OutDataTypeStr=Inherit: Same as first input
  Saturation : Saturate  UpperLimit=1  LowerLimit=-1
  Sum : Sum  Inputs=+-  SaturateOnIntegerOverflow=on  InputSameDT=on  OutDataTypeStr=Inherit: Same as first input
  Sum1 : Sum  Inputs=++-  SaturateOnIntegerOverflow=on  InputSameDT=on  OutDataTypeStr=Inherit: Same as first input
  Position : Outport
  wires:
  Gear/1 -> Conversion Rad to Deg/1
  Sum1/1 -> Gear/1
  Sum/1 -> Product/1
  Dead Zone/1 -> Saturation/1
  Derivative/1 -> Dead Zone/1
  Mux/1 -> Atan2/1
  Sin/1 -> Mux/1
  Conversion Rad to Deg/1 -> Position/1
  Saturation/1 -> Sum/2
  Conversion Rotation to Angle/1 -> Sum1/1
  Reset (Impulse)/1 -> Product/2, Init Angle/2
  Atan2/1 -> Derivative/1, Sum1/2, Init Angle/3
  Cos/1 -> Mux/2
  Memory/1 -> Sum/1
  Product/1 -> Conversion Rotation to Angle/1, Memory/1
  Memory1/1 -> Init Angle/1
  Init Angle/1 -> Sum1/3, Memory1/1

== system IRP6/Position 2/Filters 2 ==
  Sin && Cos : Inport
  Analog Butterworth LP Filter : Subsystem  mask(buttap){Parameter1=2*pi*16, Parameter2=1}
      mask prompts: Parameter1 "Cutoff frequency (rad/sec)"; Parameter2 "Order"
      mask help:
      | Analog Butterworth low pass filter.
      |
      | (Requires Signal Processing Toolbox)
      mask init:
      | [z,p,k]=buttap(@2); z=@1*z; p=@1*p; k=real(prod(-p)); [num,den]=zp2tf(z,p,k); w=logspace(log10(@1/10),log10(10*@1),20); h=freqs(num,den,w);
      mask Help: Butterworth low pass filter using MATLAB's butter command.
      mask Display: plot(20*log10(w),20*log10(abs(h)))
  Analog Butterworth LP Filter1 : Subsystem  mask(buttap){Parameter1=2*pi*16, Parameter2=1}
      mask prompts: Parameter1 "Cutoff frequency (rad/sec)"; Parameter2 "Order"
      mask help:
      | Analog Butterworth low pass filter.
      |
      | (Requires Signal Processing Toolbox)
      mask init:
      | [z,p,k]=buttap(@2); z=@1*z; p=@1*p; k=real(prod(-p)); [num,den]=zp2tf(z,p,k); w=logspace(log10(@1/10),log10(10*@1),20); h=freqs(num,den,w);
      mask Help: Butterworth low pass filter using MATLAB's butter command.
      mask Display: plot(20*log10(w),20*log10(abs(h)))
  Demux : Demux  Outputs=2
  Sin : Outport
  Cos : Outport  Port=2
  wires:
  Analog Butterworth LP Filter/1(Out1) -> Sin/1
  Analog Butterworth LP Filter1/1(Out1) -> Cos/1
  Sin && Cos/1 -> Demux/1
  Demux/1 -> Analog Butterworth LP Filter/1(In1)
  Demux/2 -> Analog Butterworth LP Filter1/1(In1)

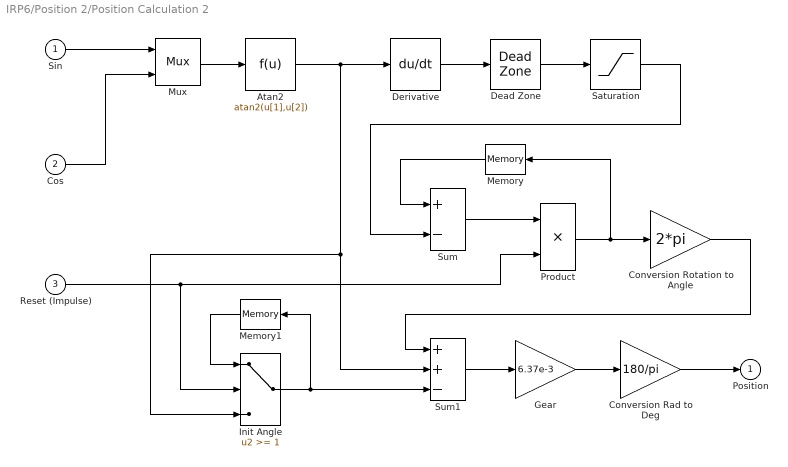
== system IRP6/Position 2/Position Calculation 2 ==
  Sin : Inport
  Cos : Inport  Port=2
  Reset (Impulse) : Inport  Port=3
  Atan2 : Fcn  Expr=atan2(u[1],u[2])
  Conversion Rad to Deg : Gain  Gain=180/pi  SaturateOnIntegerOverflow=on  OutDataTypeStr=Inherit: Same as input  ParamDataTypeStr=Inherit: Same as input
  Conversion Rotation to Angle : Gain  Gain=2*pi  SaturateOnIntegerOverflow=on  OutDataTypeStr=Inherit: Same as input  ParamDataTypeStr=Inherit: Same as input
  Dead Zone : DeadZone  LowerValue=-5000  UpperValue=5000  SaturateOnIntegerOverflow=on
  Derivative : Derivative
  Gear : Gain  Gain=6.37e-3  SaturateOnIntegerOverflow=on  OutDataTypeStr=Inherit: Same as input  ParamDataTypeStr=Inherit: Same as input
  Init Angle : Switch  Threshold=1  SaturateOnIntegerOverflow=on  InputSameDT=on
  Memory : Memory
  Memory1 : Memory
  Mux : Mux  Inputs=2
  Product : Product  SaturateOnIntegerOverflow=on  RndMeth=Zero  InputSameDT=on  OutDataTypeStr=Inherit: Same as first input
  Saturation : Saturate  UpperLimit=1  LowerLimit=-1
  Sum : Sum  Inputs=+-  SaturateOnIntegerOverflow=on  InputSameDT=on  OutDataTypeStr=Inherit: Same as first input
  Sum1 : Sum  Inputs=++-  SaturateOnIntegerOverflow=on  InputSameDT=on  OutDataTypeStr=Inherit: Same as first input
  Position : Outport
  wires:
  Gear/1 -> Conversion Rad to Deg/1
  Sum1/1 -> Gear/1
  Sum/1 -> Product/1
  Dead Zone/1 -> Saturation/1
  Derivative/1 -> Dead Zone/1
  Mux/1 -> Atan2/1
  Sin/1 -> Mux/1
  Conversion Rad to Deg/1 -> Position/1
  Saturation/1 -> Sum/2
  Conversion Rotation to Angle/1 -> Sum1/1
  Reset (Impulse)/1 -> Product/2, Init Angle/2
  Atan2/1 -> Derivative/1, Sum1/2, Init Angle/3
  Cos/1 -> Mux/2
  Memory/1 -> Sum/1
  Product/1 -> Conversion Rotation to Angle/1, Memory/1
  Memory1/1 -> Init Angle/1
  Init Angle/1 -> Sum1/3, Memory1/1

== system IRP6/Position 3/Filters 3 ==
  Sin && Cos : Inport
  Analog Butterworth LP Filter : Subsystem  mask(buttap){Parameter1=2*pi*16, Parameter2=1}
      mask prompts: Parameter1 "Cutoff frequency (rad/sec)"; Parameter2 "Order"
      mask help:
      | Analog Butterworth low pass filter.
      |
      | (Requires Signal Processing Toolbox)
      mask init:
      | [z,p,k]=buttap(@2); z=@1*z; p=@1*p; k=real(prod(-p)); [num,den]=zp2tf(z,p,k); w=logspace(log10(@1/10),log10(10*@1),20); h=freqs(num,den,w);
      mask Help: Butterworth low pass filter using MATLAB's butter command.
      mask Display: plot(20*log10(w),20*log10(abs(h)))
  Analog Butterworth LP Filter1 : Subsystem  mask(buttap){Parameter1=2*pi*16, Parameter2=1}
      mask prompts: Parameter1 "Cutoff frequency (rad/sec)"; Parameter2 "Order"
      mask help:
      | Analog Butterworth low pass filter.
      |
      | (Requires Signal Processing Toolbox)
      mask init:
      | [z,p,k]=buttap(@2); z=@1*z; p=@1*p; k=real(prod(-p)); [num,den]=zp2tf(z,p,k); w=logspace(log10(@1/10),log10(10*@1),20); h=freqs(num,den,w);
      mask Help: Butterworth low pass filter using MATLAB's butter command.
      mask Display: plot(20*log10(w),20*log10(abs(h)))
  Demux : Demux  Outputs=2
  Sin : Outport
  Cos : Outport  Port=2
  wires:
  Analog Butterworth LP Filter/1(Out1) -> Sin/1
  Analog Butterworth LP Filter1/1(Out1) -> Cos/1
  Sin && Cos/1 -> Demux/1
  Demux/1 -> Analog Butterworth LP Filter/1(In1)
  Demux/2 -> Analog Butterworth LP Filter1/1(In1)

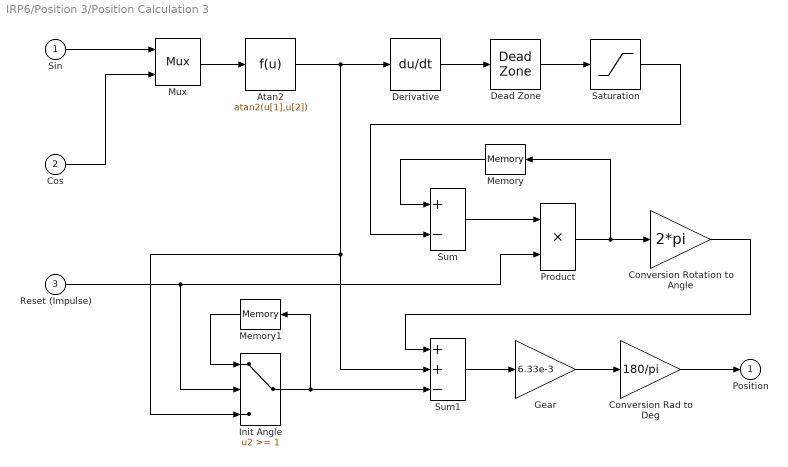
== system IRP6/Position 3/Position Calculation 3 ==
  Sin : Inport
  Cos : Inport  Port=2
  Reset (Impulse) : Inport  Port=3
  Atan2 : Fcn  Expr=atan2(u[1],u[2])
  Conversion Rad to Deg : Gain  Gain=180/pi  SaturateOnIntegerOverflow=on  OutDataTypeStr=Inherit: Same as input  ParamDataTypeStr=Inherit: Same as input
  Conversion Rotation to Angle : Gain  Gain=2*pi  SaturateOnIntegerOverflow=on  OutDataTypeStr=Inherit: Same as input  ParamDataTypeStr=Inherit: Same as input
  Dead Zone : DeadZone  LowerValue=-5000  UpperValue=5000  SaturateOnIntegerOverflow=on
  Derivative : Derivative
  Gear : Gain  Gain=6.33e-3  SaturateOnIntegerOverflow=on  OutDataTypeStr=Inherit: Same as input  ParamDataTypeStr=Inherit: Same as input
  Init Angle : Switch  Threshold=1  SaturateOnIntegerOverflow=on  InputSameDT=on
  Memory : Memory
  Memory1 : Memory
  Mux : Mux  Inputs=2
  Product : Product  SaturateOnIntegerOverflow=on  RndMeth=Zero  InputSameDT=on  OutDataTypeStr=Inherit: Same as first input
  Saturation : Saturate  UpperLimit=1  LowerLimit=-1
  Sum : Sum  Inputs=+-  SaturateOnIntegerOverflow=on  InputSameDT=on  OutDataTypeStr=Inherit: Same as first input
  Sum1 : Sum  Inputs=++-  SaturateOnIntegerOverflow=on  InputSameDT=on  OutDataTypeStr=Inherit: Same as first input
  Position : Outport
  wires:
  Gear/1 -> Conversion Rad to Deg/1
  Sum1/1 -> Gear/1
  Sum/1 -> Product/1
  Dead Zone/1 -> Saturation/1
  Derivative/1 -> Dead Zone/1
  Mux/1 -> Atan2/1
  Sin/1 -> Mux/1
  Conversion Rad to Deg/1 -> Position/1
  Saturation/1 -> Sum/2
  Conversion Rotation to Angle/1 -> Sum1/1
  Reset (Impulse)/1 -> Product/2, Init Angle/2
  Atan2/1 -> Derivative/1, Sum1/2, Init Angle/3
  Cos/1 -> Mux/2
  Memory/1 -> Sum/1
  Product/1 -> Conversion Rotation to Angle/1, Memory/1
  Memory1/1 -> Init Angle/1
  Init Angle/1 -> Sum1/3, Memory1/1

== system IRP6/Position 4/Filters 4 ==
  Sin && Cos : Inport
  Analog Butterworth LP Filter : Subsystem  mask(buttap){Parameter1=2*pi*16, Parameter2=1}
      mask prompts: Parameter1 "Cutoff frequency (rad/sec)"; Parameter2 "Order"
      mask help:
      | Analog Butterworth low pass filter.
      |
      | (Requires Signal Processing Toolbox)
      mask init:
      | [z,p,k]=buttap(@2); z=@1*z; p=@1*p; k=real(prod(-p)); [num,den]=zp2tf(z,p,k); w=logspace(log10(@1/10),log10(10*@1),20); h=freqs(num,den,w);
      mask Help: Butterworth low pass filter using MATLAB's butter command.
      mask Display: plot(20*log10(w),20*log10(abs(h)))
  Analog Butterworth LP Filter1 : Subsystem  mask(buttap){Parameter1=2*pi*16, Parameter2=1}
      mask prompts: Parameter1 "Cutoff frequency (rad/sec)"; Parameter2 "Order"
      mask help:
      | Analog Butterworth low pass filter.
      |
      | (Requires Signal Processing Toolbox)
      mask init:
      | [z,p,k]=buttap(@2); z=@1*z; p=@1*p; k=real(prod(-p)); [num,den]=zp2tf(z,p,k); w=logspace(log10(@1/10),log10(10*@1),20); h=freqs(num,den,w);
      mask Help: Butterworth low pass filter using MATLAB's butter command.
      mask Display: plot(20*log10(w),20*log10(abs(h)))
  Demux : Demux  Outputs=2
  Sin : Outport
  Cos : Outport  Port=2
  wires:
  Demux/2 -> Analog Butterworth LP Filter1/1(In1)
  Demux/1 -> Analog Butterworth LP Filter/1(In1)
  Sin && Cos/1 -> Demux/1
  Analog Butterworth LP Filter1/1(Out1) -> Cos/1
  Analog Butterworth LP Filter/1(Out1) -> Sin/1

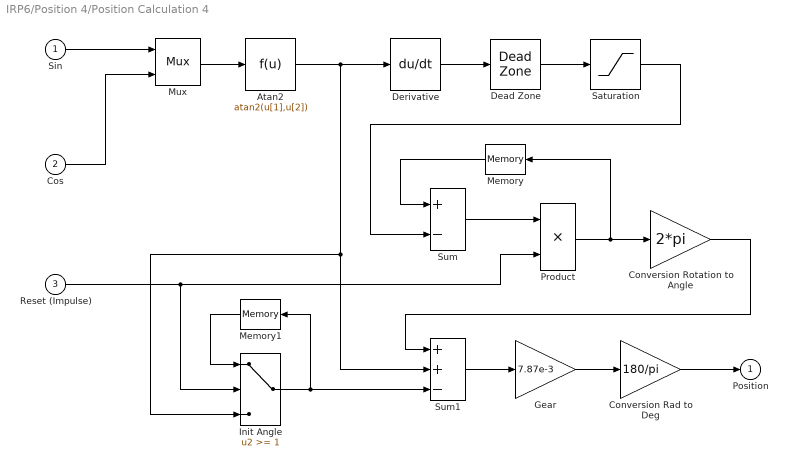
== system IRP6/Position 4/Position Calculation 4 ==
  Sin : Inport
  Cos : Inport  Port=2
  Reset (Impulse) : Inport  Port=3
  Atan2 : Fcn  Expr=atan2(u[1],u[2])
  Conversion Rad to Deg : Gain  Gain=180/pi  SaturateOnIntegerOverflow=on  OutDataTypeStr=Inherit: Same as input  ParamDataTypeStr=Inherit: Same as input
  Conversion Rotation to Angle : Gain  Gain=2*pi  SaturateOnIntegerOverflow=on  OutDataTypeStr=Inherit: Same as input  ParamDataTypeStr=Inherit: Same as input
  Dead Zone : DeadZone  LowerValue=-5000  UpperValue=5000  SaturateOnIntegerOverflow=on
  Derivative : Derivative
  Gear : Gain  Gain=7.87e-3  SaturateOnIntegerOverflow=on  OutDataTypeStr=Inherit: Same as input  ParamDataTypeStr=Inherit: Same as input
  Init Angle : Switch  Threshold=1  SaturateOnIntegerOverflow=on  InputSameDT=on
  Memory : Memory
  Memory1 : Memory
  Mux : Mux  Inputs=2
  Product : Product  SaturateOnIntegerOverflow=on  RndMeth=Zero  InputSameDT=on  OutDataTypeStr=Inherit: Same as first input
  Saturation : Saturate  UpperLimit=1  LowerLimit=-1
  Sum : Sum  Inputs=+-  SaturateOnIntegerOverflow=on  InputSameDT=on  OutDataTypeStr=Inherit: Same as first input
  Sum1 : Sum  Inputs=++-  SaturateOnIntegerOverflow=on  InputSameDT=on  OutDataTypeStr=Inherit: Same as first input
  Position : Outport
  wires:
  Init Angle/1 -> Memory1/1, Sum1/3
  Memory1/1 -> Init Angle/1
  Product/1 -> Memory/1, Conversion Rotation to Angle/1
  Memory/1 -> Sum/1
  Cos/1 -> Mux/2
  Atan2/1 -> Init Angle/3, Sum1/2, Derivative/1
  Reset (Impulse)/1 -> Init Angle/2, Product/2
  Conversion Rotation to Angle/1 -> Sum1/1
  Saturation/1 -> Sum/2
  Conversion Rad to Deg/1 -> Position/1
  Sin/1 -> Mux/1
  Mux/1 -> Atan2/1
  Derivative/1 -> Dead Zone/1
  Dead Zone/1 -> Saturation/1
  Sum/1 -> Product/1
  Sum1/1 -> Gear/1
  Gear/1 -> Conversion Rad to Deg/1

== system IRP6/Position 5/Filters 5 ==
  Sin && Cos : Inport
  Analog Butterworth LP Filter : Subsystem  mask(buttap){Parameter1=2*pi*16, Parameter2=1}
      mask prompts: Parameter1 "Cutoff frequency (rad/sec)"; Parameter2 "Order"
      mask help:
      | Analog Butterworth low pass filter.
      |
      | (Requires Signal Processing Toolbox)
      mask init:
      | [z,p,k]=buttap(@2); z=@1*z; p=@1*p; k=real(prod(-p)); [num,den]=zp2tf(z,p,k); w=logspace(log10(@1/10),log10(10*@1),20); h=freqs(num,den,w);
      mask Help: Butterworth low pass filter using MATLAB's butter command.
      mask Display: plot(20*log10(w),20*log10(abs(h)))
  Analog Butterworth LP Filter1 : Subsystem  mask(buttap){Parameter1=2*pi*16, Parameter2=1}
      mask prompts: Parameter1 "Cutoff frequency (rad/sec)"; Parameter2 "Order"
      mask help:
      | Analog Butterworth low pass filter.
      |
      | (Requires Signal Processing Toolbox)
      mask init:
      | [z,p,k]=buttap(@2); z=@1*z; p=@1*p; k=real(prod(-p)); [num,den]=zp2tf(z,p,k); w=logspace(log10(@1/10),log10(10*@1),20); h=freqs(num,den,w);
      mask Help: Butterworth low pass filter using MATLAB's butter command.
      mask Display: plot(20*log10(w),20*log10(abs(h)))
  Demux : Demux  Outputs=2
  Sin : Outport
  Cos : Outport  Port=2
  wires:
  Demux/2 -> Analog Butterworth LP Filter1/1(In1)
  Demux/1 -> Analog Butterworth LP Filter/1(In1)
  Sin && Cos/1 -> Demux/1
  Analog Butterworth LP Filter1/1(Out1) -> Cos/1
  Analog Butterworth LP Filter/1(Out1) -> Sin/1

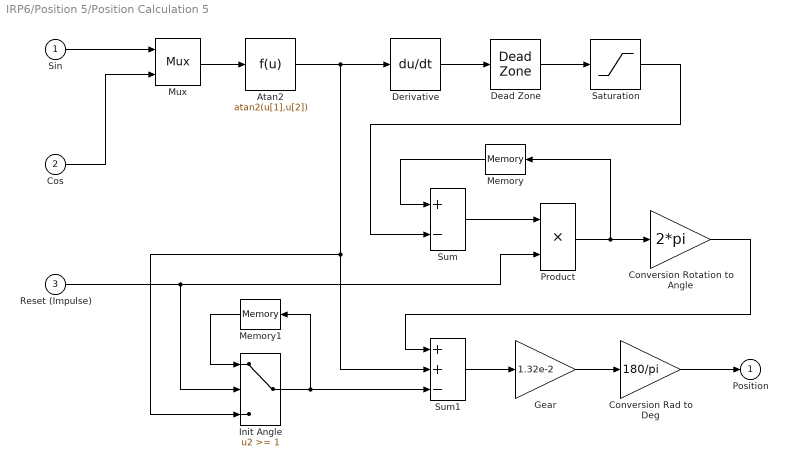
== system IRP6/Position 5/Position Calculation 5 ==
  Sin : Inport
  Cos : Inport  Port=2
  Reset (Impulse) : Inport  Port=3
  Atan2 : Fcn  Expr=atan2(u[1],u[2])
  Conversion Rad to Deg : Gain  Gain=180/pi  SaturateOnIntegerOverflow=on  OutDataTypeStr=Inherit: Same as input  ParamDataTypeStr=Inherit: Same as input
  Conversion Rotation to Angle : Gain  Gain=2*pi  SaturateOnIntegerOverflow=on  OutDataTypeStr=Inherit: Same as input  ParamDataTypeStr=Inherit: Same as input
  Dead Zone : DeadZone  LowerValue=-5000  UpperValue=5000  SaturateOnIntegerOverflow=on
  Derivative : Derivative
  Gear : Gain  Gain=1.32e-2  SaturateOnIntegerOverflow=on  OutDataTypeStr=Inherit: Same as input  ParamDataTypeStr=Inherit: Same as input
  Init Angle : Switch  Threshold=1  SaturateOnIntegerOverflow=on  InputSameDT=on
  Memory : Memory
  Memory1 : Memory
  Mux : Mux  Inputs=2
  Product : Product  SaturateOnIntegerOverflow=on  RndMeth=Zero  InputSameDT=on  OutDataTypeStr=Inherit: Same as first input
  Saturation : Saturate  UpperLimit=1  LowerLimit=-1
  Sum : Sum  Inputs=+-  SaturateOnIntegerOverflow=on  InputSameDT=on  OutDataTypeStr=Inherit: Same as first input
  Sum1 : Sum  Inputs=++-  SaturateOnIntegerOverflow=on  InputSameDT=on  OutDataTypeStr=Inherit: Same as first input
  Position : Outport
  wires:
  Init Angle/1 -> Memory1/1, Sum1/3
  Memory1/1 -> Init Angle/1
  Product/1 -> Memory/1, Conversion Rotation to Angle/1
  Memory/1 -> Sum/1
  Cos/1 -> Mux/2
  Atan2/1 -> Init Angle/3, Sum1/2, Derivative/1
  Reset (Impulse)/1 -> Init Angle/2, Product/2
  Conversion Rotation to Angle/1 -> Sum1/1
  Saturation/1 -> Sum/2
  Conversion Rad to Deg/1 -> Position/1
  Sin/1 -> Mux/1
  Mux/1 -> Atan2/1
  Derivative/1 -> Dead Zone/1
  Dead Zone/1 -> Saturation/1
  Sum/1 -> Product/1
  Sum1/1 -> Gear/1
  Gear/1 -> Conversion Rad to Deg/1
